simulink model "generate_elbow_motion"  (R2023a)
settings: Solver=FixedStepDiscrete  StartTime=0.0  StopTime=inf  FixedStep=0.001  RelTol=1e-3  EnableMultiTasking=on
PreLoadFcn:
  | frs = FrankaRobotSettings();
libraries: franka_simulink_library x4
settings Model: SimulationMode=external  ExtModeTrigDuration=10000  Creator=vasi_ko  LastModifiedBy=kvasios
settings SolverCC: AlgebraicLoopSolver=TrustRegion
settings DataIOCC: LimitDataPoints=on  SaveFormat=Array  ReturnWorkspaceOutputs=off
settings OptimizationCC: DefaultParameterBehavior=Inlined  EnhancedBackFolding=on  PassReuseOutputArgsThreshold=0  OptimizeBlockOrder=speed  DifferentSizesBufferReuse=on  OptimizationCustomize=off
settings DebuggingCC: SolverPrmCheckMsg=warning  ParameterTunabilityLossMsg=error  UnconnectedInputMsg=warning  UnconnectedOutputMsg=warning  UnconnectedLineMsg=warning  SFUnexpectedBacktrackingDiag=warning  SFNoUnconditionalDefaultTransitionDiag=warning  SFExecutionAtInitializationDiag=none  ArithmeticOperatorsInVariantConditions=warning
settings ModelReferenceCC: EnableRefExpFcnMdlSchedulingChecks=on  PropagateSignalLabelsOutOfModel=off
settings SFSimCC: SimUseLocalCustomCode=off  MATLABDynamicMemAlloc=off  CustomCodeUndefinedFunction=UseInterfaceOnly  SimTargetLang=C++
settings RTWCC: RTWVerbose=off  RTWUseLocalCustomCode=off  BuildConfiguration=Faster Runs  TargetLang=C++  DLArmComputeVersion=19.05
settings CodeAppCC: ForceParamTrailComments=on  OperatorAnnotations=on
settings ConfigComp: CovMetricSettings=dw  CovSaveCumulativeToWorkspaceVar=on  CovSaveSingleToWorkspaceVar=on  CovExternalEMLEnable=off  CovSFcnEnable=off

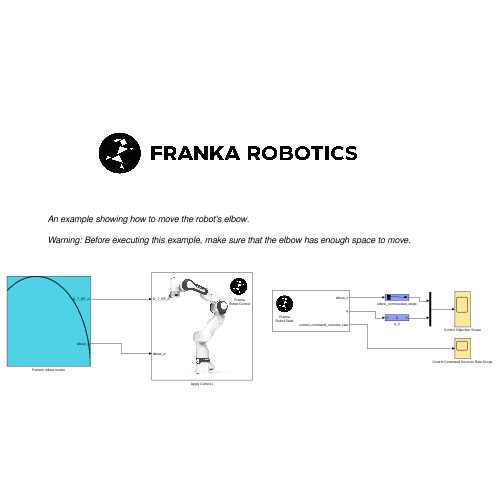
[thumbnail: Simulink's stored preview of the top-level diagram]
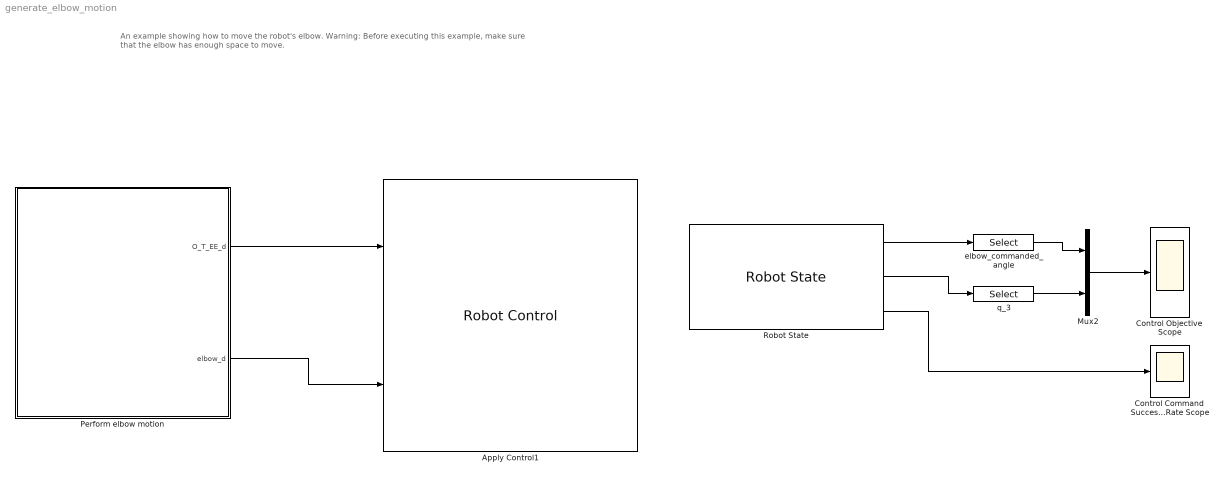
== system generate_elbow_motion ==
  note: An example showing how to move the robot's elbow.
      |
      | Warning: Before executing this example, make sure that the elbow has enough space to move.
  Apply Control1 : franka_simulink_library/Robot Control  robot_ip=frs.robot_ip  gripper_selection=None  control_mode=Cartesian Pose - Internal Controller Mode  controller_choice=Joint Impedance Controller  joint_impedance=frs.joint_impedance_stiffness  cartesian_impedance=[3000, 3000, 3000, 300, 300, 300]  rate_limiter=on  cuttoff_frequency=frs.cutoff_frequency  elbow_control=on  collision_thresholds=frs.collision_thresholds.getAs1DArray  load_inertia=frs.load_inertia.getAs1DArray  NE_T_EE=frs.NE_T_EE(:)  EE_T_K=frs.EE_T_K(:)  init_joint_configuration_req=on  init_joint_configuration=frs.home_configuration
      settings: SourceProductName=Franka Robotics Simulink Support Package
  Control Command Success Rate Scope : Scope
  Control Objective Scope : Scope
  Mux2 : Mux  Inputs=2
  Perform elbow motion : Subsystem
      mask Display:
      | pos = get_param(gcb, 'Position');
      | width = pos(3) - pos(1);
      | x = [0:width];
      | y = sin(x/180*pi);
      | % Parameters 'm' and 'b' must be defined in 'Parameters & Dialog' pane.
      | plot(cos(x/180*pi*0.5), sin(x/180*pi*0.5));
      | 
      | port_label('output',1,'O_T_EE_d');
      | port_label('output',2,'elbow_d');
  Robot State : franka_simulink_library/Robot State  robot_ip=frs.robot_ip  signals_requested='elbow_c q control_command_success_rate'
      settings: SourceProductName=Franka Robotics Simulink Support Package
  elbow_commanded_angle : Selector  InputPortWidth=2  IndexOptions=Index vector (dialog)  Indices=1  OutputSizes=1
  q_3 : Selector  InputPortWidth=7  IndexOptions=Index vector (dialog)  Indices=3  OutputSizes=1
  wires:
  Perform elbow motion/1(O_T_EE_d) -> Apply Control1/1
  Robot State/1 -> elbow_commanded_angle/1
  Robot State/2 -> q_3/1
  Mux2/1 -> Control Objective Scope/1
  elbow_commanded_angle/1 -> Mux2/1
  q_3/1 -> Mux2/2
  Robot State/3 -> Control Command Success Rate Scope/1
  Perform elbow motion/2(elbow_d) -> Apply Control1/2

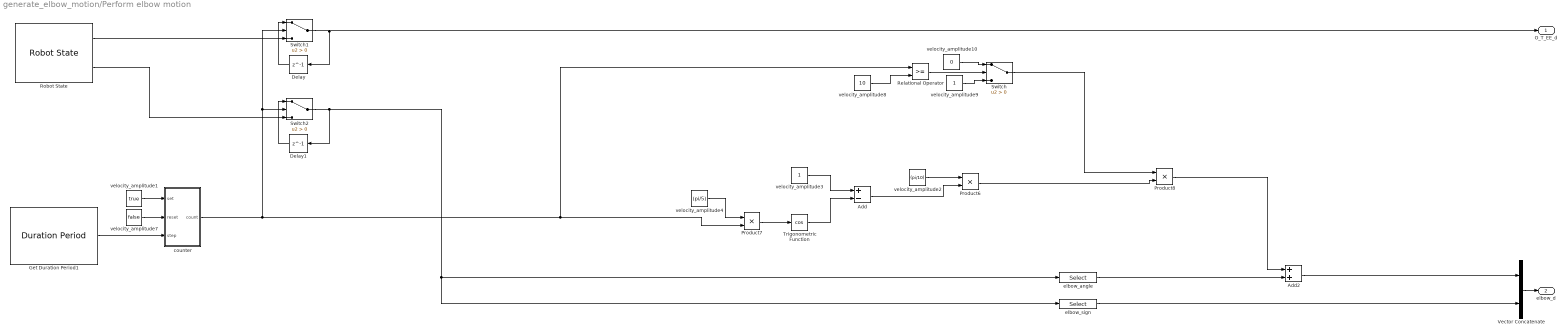
== system generate_elbow_motion/Perform elbow motion ==
  Add : Sum  Inputs=+-
  Add2 : Sum
  Delay : Delay  DelayLength=1
  Delay1 : Delay  DelayLength=1
  Get Duration Period1 : franka_simulink_library/Duration Period  robot_ip=frs.robot_ip
      settings: SourceProductName=Franka Robotics Simulink Support Package
  Product6 : Product
  Product7 : Product
  Product8 : Product
  Relational Operator : RelationalOperator  OutDataTypeStr=boolean  InputSameDT=off
  Robot State : franka_simulink_library/Robot State  robot_ip=frs.robot_ip  signals_requested='O_T_EE_c elbow_c'
      settings: SourceProductName=Franka Robotics Simulink Support Package
  Switch : Switch  Criteria=u2 > Threshold  SaturateOnIntegerOverflow=off  InputSameDT=off
  Switch1 : Switch  Criteria=u2 > Threshold  SaturateOnIntegerOverflow=off  InputSameDT=off
  Switch2 : Switch  Criteria=u2 > Threshold  SaturateOnIntegerOverflow=off  InputSameDT=off
  Trigonometric Function : Trigonometry  Operator=cos  NumberOfIterations=50
  Vector Concatenate : Concatenate
  counter : Subsystem
  elbow_angle : Selector  InputPortWidth=2  IndexOptions=Index vector (dialog)  Indices=1  OutputSizes=1
  elbow_sign : Selector  InputPortWidth=2  IndexOptions=Index vector (dialog)  Indices=2  OutputSizes=1
  velocity_amplitude1 : Constant  Value=true  VectorParams1D=off
  velocity_amplitude10 : Constant  Value=0  VectorParams1D=off
  velocity_amplitude2 : Constant  Value=(pi/10)  VectorParams1D=off
  velocity_amplitude3 : Constant  VectorParams1D=off
  velocity_amplitude4 : Constant  Value=(pi/5)  VectorParams1D=off
  velocity_amplitude7 : Constant  Value=false  VectorParams1D=off
  velocity_amplitude8 : Constant  Value=10  VectorParams1D=off
  velocity_amplitude9 : Constant  VectorParams1D=off
  O_T_EE_d : Outport  VectorParamsAs1DForOutWhenUnconnected=off
  elbow_d : Outport  Port=2  VectorParamsAs1DForOutWhenUnconnected=off
  wires:
  Product8/1 -> Add2/1
  elbow_angle/1 -> Add2/2
  Switch2/1 -> elbow_angle/1, elbow_sign/1, Delay1/1
  velocity_amplitude2/1 -> Product6/1
  velocity_amplitude3/1 -> Add/1
  velocity_amplitude4/1 -> Product7/1
  Trigonometric Function/1 -> Add/2
  Product7/1 -> Trigonometric Function/1
  Add/1 -> Product6/2
  Switch/1 -> Product8/1
  Get Duration Period1/1 -> counter/3(step)
  velocity_amplitude1/1 -> counter/1(set)
  velocity_amplitude7/1 -> counter/2(reset)
  velocity_amplitude8/1 -> Relational Operator/2
  Relational Operator/1 -> Switch/2
  velocity_amplitude9/1 -> Switch/3
  velocity_amplitude10/1 -> Switch/1
  Switch1/1 -> O_T_EE_d/1, Delay/1
  Vector Concatenate/1 -> elbow_d/1
  Add2/1 -> Vector Concatenate/1
  elbow_sign/1 -> Vector Concatenate/2
  Product6/1 -> Product8/2
  Delay/1 -> Switch1/1
  Delay1/1 -> Switch2/1
  counter/1(count) -> Relational Operator/1, Product7/2, Switch1/2, Switch2/2
  Robot State/2 -> Switch2/3
  Robot State/1 -> Switch1/3

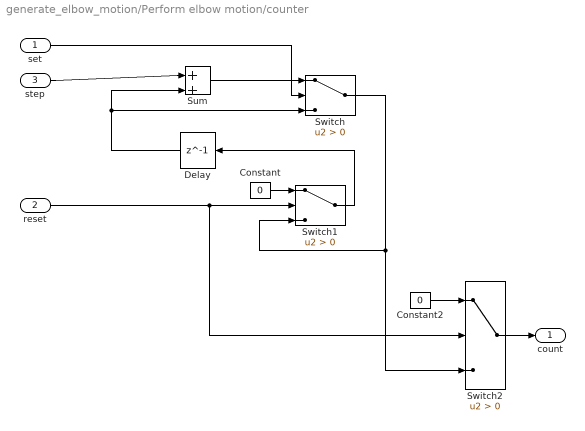
== system generate_elbow_motion/Perform elbow motion/counter ==
  set : Inport  OutDataTypeStr=boolean
  reset : Inport  Port=2  OutDataTypeStr=boolean
  step : Inport  Port=3  OutDataTypeStr=double
  Constant : Constant  Value=0  OutDataTypeStr=double
  Constant2 : Constant  Value=0  OutDataTypeStr=double
  Delay : Delay  DelayLength=1  InitialCondition=0
  Sum : Sum  Inputs=|++
  Switch : Switch  Criteria=u2 > Threshold  SaturateOnIntegerOverflow=off  InputSameDT=off
  Switch1 : Switch  Criteria=u2 > Threshold  OutDataTypeStr=double  SaturateOnIntegerOverflow=off  InputSameDT=off
  Switch2 : Switch  Criteria=u2 > Threshold  OutDataTypeStr=double  SaturateOnIntegerOverflow=off  InputSameDT=off
  count : Outport  OutDataTypeStr=double  VectorParamsAs1DForOutWhenUnconnected=off
  wires:
  Switch1/1 -> Delay/1
  Constant/1 -> Switch1/1
  reset/1 -> Switch2/2, Switch1/2
  Delay/1 -> Switch/3, Sum/2
  step/1 -> Sum/1
  Switch/1 -> Switch2/3, Switch1/3
  set/1 -> Switch/2
  Sum/1 -> Switch/1
  Constant2/1 -> Switch2/1
  Switch2/1 -> count/1
